simulink model "test_small_model"  (R2021b)
settings: Solver=VariableStepAuto  StartTime=0.0  StopTime=40  RelTol=1e-3
values from neighbouring files (symbols this model uses):
  A = J    (= 0.066829)    [test_big.m]    (also in test_small.m = 0.000254045)
  B = b_m + b + (b/(N^2*n_g))    (= 0.00010739)    [test_big.m]    (also in test_small.m = 6e-07)
  D = (mu_s*cos(angl) + sin(angl)) * r_p*(m_l+m_b)*g/(N*n_g)    [test_big.m]    (also in test_small.m = 0.113379075)
  Ke = 0.0537    [test_big.m]    (also in test_small.m = 0.0168)
  N = (1:0.1:50)    [gear_ratio_code_1.m]    (also in test_big.m = 1; test_small.m = 1)
  R = 0.0821    [test_big.m]    (also in test_small.m = 3.17)
  r_p = 0.5e-1    (= 0.05)    [test_big.m]    (also in test_small.m = 0.005)
  V = 24    [test_big.m]    (also in test_small.m = 12)
undefined symbols (not defined in the file or in its folder): Tm
settings Model: Creator=marcelafunyah  LastModifiedBy=marcelafunyah

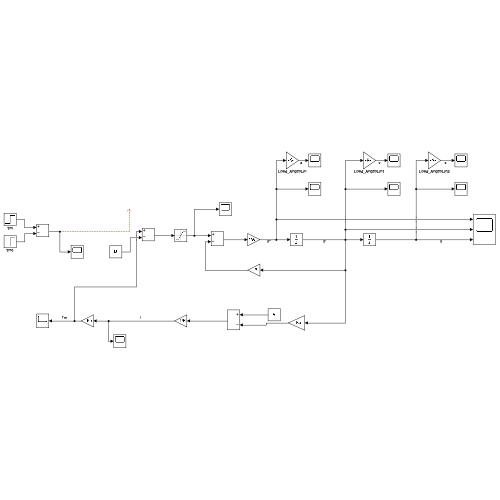
[thumbnail: Simulink's stored preview of the top-level diagram]
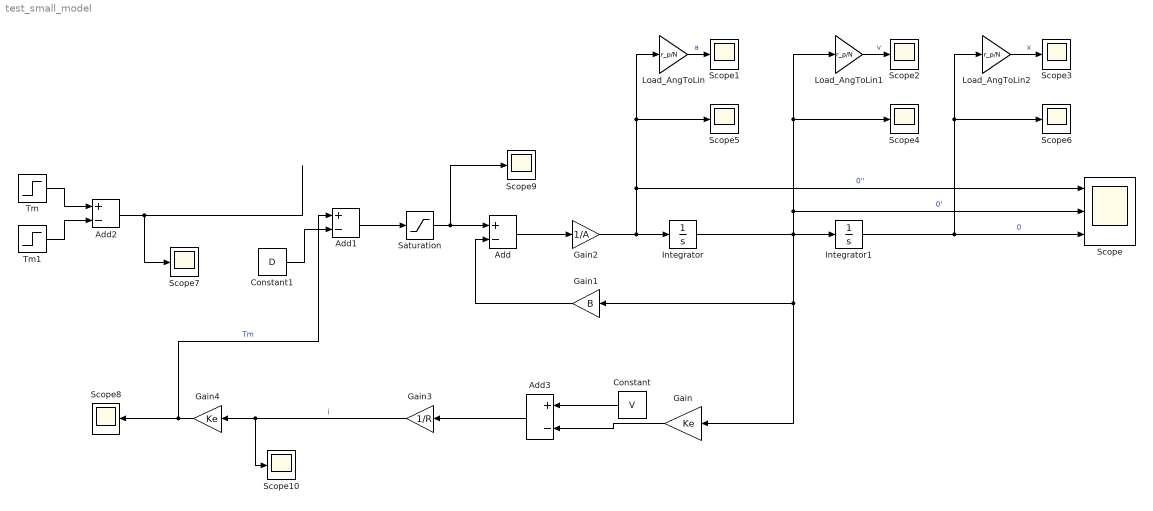
== system test_small_model ==
  Add{,1..3} (4 alike) : Sum  Inputs=+-
  Constant : Constant  Value=V
  Constant1 : Constant  Value=D
  Gain : Gain  Gain=Ke
  Gain1 : Gain  Gain=B
  Gain2 : Gain  Gain=1/A
  Gain3 : Gain  Gain=1/R
  Gain4 : Gain  Gain=Ke
  Integrator : Integrator
  Integrator1 : Integrator
  Load_AngToLin : Gain  Gain=r_p/N
  Load_AngToLin1 : Gain  Gain=r_p/N
  Load_AngToLin2 : Gain  Gain=r_p/N
  Saturation : Saturate  UpperLimit=9999999999  LowerLimit=0
  Scope : Scope  NumInputPorts=3
  Scope{1..10} (10 alike) : Scope
  Tm : Step  Time=0  After=Tm  SampleTime=0
  Tm1 : Step  Time=15  After=Tm  SampleTime=0
  wires:
  Integrator/1 -> Scope4/1, Load_AngToLin1/1, Scope/2, Gain1/1, Gain/1, Integrator1/1  "0'"
  Integrator1/1 -> Load_AngToLin2/1, Scope6/1, Scope/3  "0"
  Gain2/1 -> Scope5/1, Load_AngToLin/1, Scope/1, Integrator/1  "0''"
  Gain1/1 -> Add/2
  Load_AngToLin/1 -> Scope1/1  "a"
  Load_AngToLin1/1 -> Scope2/1  "v"
  Load_AngToLin2/1 -> Scope3/1  "x"
  Add/1 -> Gain2/1
  Constant1/1 -> Add1/2
  Saturation/1 -> Scope9/1, Add/1
  Add1/1 -> Saturation/1
  Tm/1 -> Add2/1
  Tm1/1 -> Add2/2
  Add2/1 -> Scope7/1
  Constant/1 -> Add3/1
  Gain/1 -> Add3/2
  Add3/1 -> Gain3/1
  Gain3/1 -> Scope10/1, Gain4/1  "i"
  Gain4/1 -> Add1/1, Scope8/1  "Tm"
